simulink model "Simulink"  (Simulink 8.7)
settings: Solver=ode45  StartTime=0.0  StopTime=40  RelTol=1e-3
settings Model: Creator=allen  LastModifiedBy=Allen Hichard
settings DebuggingCC: UnderspecifiedInitializationDetection=Simplified  MergeDetectMultiDrivingBlocksExec=error

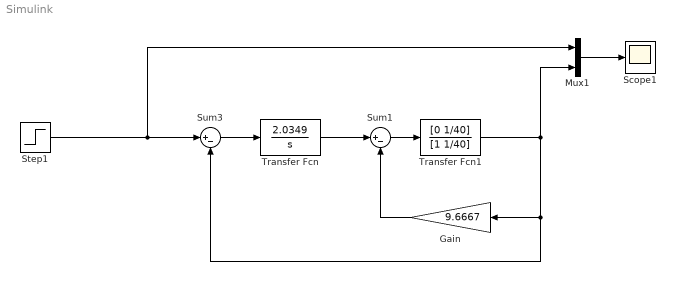
== system Simulink ==
  Gain : Gain  Gain=9.6667
  Mux1 : Mux  Inputs=2
  Scope1 : Scope
  Step1 : Step  SampleTime=0
  Sum1 : Sum  Inputs=|+-
  Sum3 : Sum  Inputs=|+-
  Transfer Fcn : TransferFcn  Numerator=[2.0349]  Denominator=[1 0]
  Transfer Fcn1 : TransferFcn  Numerator=[0 1/40]  Denominator=[1 1/40]
  wires:
  Mux1/1 -> Scope1/1
  Step1/1 -> Sum3/1, Mux1/1
  Sum1/1 -> Transfer Fcn1/1
  Transfer Fcn/1 -> Sum1/1
  Gain/1 -> Sum1/2
  Transfer Fcn1/1 -> Gain/1, Sum3/2, Mux1/2
  Sum3/1 -> Transfer Fcn/1
